simulink library "SUB_ECU_L4_MABX_HW_Interface"  (R2018a)
settings: Solver=VariableStepAuto  StartTime=0.0  StopTime=10.0  RelTol=1e-3
PostLoadFcn:
  | , if any(exist('dsrtsu_mdlpostloadfcn', 'file') == [2, 3, 6]), try dsrtsu_mdlpostloadfcn('Execute', bdroot); catch fprintf('Error in PostLoadFcn (dsrtsu_mdlpostloadfcn) for model "%s":\n %s\n', bdroot, lasterr); end, end,
undefined symbols (not defined in the file or in its folder): CANR_PROPB_REAX_3_13_CHANNEL_APV, CANR_PROPB_REAX_4_13_CHANNEL_APV, CANR_PROPB_XPR_1_50_CHANNEL_APV, ENUM_CAN_RX_T, ENUM_CAN_TX_T, ENUM_REAX_OPERATION_MODE_T, ENUM_SIGNAL_HEALTH_T, ENUM_XBR_CONTROL_MODE_T, ENUM_XBR_EBI_MODE_T, ENUM_XBR_PASS_THROUGH_ACTIVE_T, ENUM_XBR_PRIORITY_T, ENUM_XPR_INHIBIT_PARK_MANUAL_T, ENUM_XPR_INHIBIT_UNPARK_MANUAL_T, ENUM_XPR_PARK_MANUAL_T, ENUM_XPR_UNPARK_MANUAL_T, PROPB_REAX_1_E4_DES_POS_SIG_SRC_APV, PROPB_REAX_1_E4_DESIRED_OPMODE_APV, PROPB_REAX_1_E4_DESIRED_POSITION_APV, ptc_matlab_lib
libraries: PTC_MBDS_LIB x264, rtican x172, EmE_MBD_Blockset x39, simulink x34, $bdroot x16, rti1401lib_dio_type4 x8, simulink_need_slupdate x7, dsa_tcpip_lib x4, rti1401lib_adc_type4 x3, rtmapslib x3, rtitasklib x3
(part 17 of 51)

== system SUB_ECU_L4_MABX_HW_Interface/CAN_PIC_KW/CAN_RX_GNSSDOPs_00/RX_CAN_4 ==
  Enable : Inport
  Bus Creator1 : BusCreator  Inputs=9
  Bus Creator3 : BusCreator  Inputs=9
  Data Type Conversion{1..2,9..10} (4 alike) : DataTypeConversion  OutDataTypeStr=double  SaturateOnIntegerOverflow=on
  Data Type Conversion3 : DataTypeConversion  OutDataTypeStr=boolean  SaturateOnIntegerOverflow=on
  Data Type Conversion8 : DataTypeConversion  OutDataTypeStr=boolean  SaturateOnIntegerOverflow=on
  GNSSDOPs_011 : rtican/RTICAN Receive (RX)   Reserved1=[]  Reserved2=[]  Reserved3=[]  Reserved4=[]  SfcnMessage=[]  Msg_Struct=[]  BoardTypeNo=[]  BoardNo=[]  ChannelNo=[]  Parameters=[]  DialogFcn=[]  UnitName=[]  Revision=[]  UnitValues=[]  DSProperties=struct('RTI',struct('Version',uint32(5),'BlockType',struct('isSLSource',uint8(1),'isSLSink',uint8(1),'isHWSource',uint8(0),'isHWSink',uint8(0),'isSetup',uint8(0),'isInline',uint8(1),'isNonInline',uint8(0),'isInterrupt',uint8(0),'isChannelwise',uint8(0)),'IOBoardType','RTICAN','UnitType','MESSAGE','Identifier','RX','DialogType','MSVC','BlockSet','RTICAN','SlaveProcessor','CAN'))  RTIBlockInterface=struct('OutputPortsWidth',int32([1 1 1 1 1 1 1 1 1]),'OutputPortsActive',[1 1 1 1 1 1 1 1 1],'OutputPortsName',{{'SID','SetMode','OpMode','HDOP_','VDOP','TDOP',['RX status'],['RX time'],['RX delta time']}},'OutputPortsDataType',{{'SS_DOUBLE','SS_DOUBLE','SS_DOUBLE','SS_DOUBLE','SS_DOUBLE','SS_DOUBLE','SS_DOUBLE','SS_DOUBLE','SS_DOUBLE'}},'OutputPortsLabel',{{'SID','SetMode','OpMode','HDOP_','VDOP','TDOP','','',''}},'OutputPortsLabelMode','ON','InputPortsWidth',int32(0),'InputPortsActive',0,'DialogFcn','rtican_message_interface_gui','BlockDisplay',{{'','center'}},'IconTransparency','on','ParameterTunableNames',{{}},'InitLevel',3,'BlockName',struct('Token',{{'GNSSDOPs_01'}}),'SampleTime',{{-1}},'TriggerPort',{{'none'}},'EnablePort',{{'yes'}})  RTIBlockParameters=struct('BoardTypeNo',{{1,'OFF',[]}},'BoardNo',{{2,'ON',[1 16]}},'ChannelNo',{{2,'ON',[1 2]}},'Parameters',{{struct('DataFileSupport',struct('DataFileSelectedMaster',1,'DataFileSelectedLocal',0,'DataFileName','c:\localdata\chris\advanced_r&d\adas\level4_rcp\truck1571\dbc\mabx_can4.dbc|','DataFileDate',{{{['10-Feb-2017 15:17:28']}}},'SelectedFile','dbc\mabx_can4.dbc'),'Options',struct('StatusSelected',1,'TimeSelected',1,'DeltaTimeSelected',1,'BytePortSelected',0,'MessageLengthSelected',0,'TriggerPort',struct('Selected',0,'TriggerType',0),'UserCoding',struct('Selected',0,'InterfaceFile','UserDecodingFile','FcnName','UserDecodeFcn','InportSelected',0,'InportWidth',1,'OutportSelected',0,'OutportWidth',1),'EnablePortSelected',1,'SignalOnPortnameSelected',1,'UseRXService',1),'Message',struct('MsgOnBlocknameSelected',1,'MsgName','GNSSDOPs_01','MsgIdFormat',1,'MsgId',435815168,'MsgLength',8,'NumSignals',6,'SampleTime',-1,'Signal',struct('SgnName',{'SID','SetMode','OpMode','HDOP_','VDOP','TDOP'},'SgnStartBit',{0,8,11,16,32,48},'SgnLength',{8,3,3,16,16,16},'SgnType',{0,0,0,0,0,0},'ModeValue',{-1,-1,-1,-1,-1,-1},'DataType',{0,0,0,1,1,1},'ByteLayout',{0,0,0,0,0,0},'Factor',{1,1,1,0.01,0.01,0.01},'Offset',{0,0,0,0,0,0},'SgnComment',{{['An upward counting number used to tie related information together between different PGNs.For example,SID would be used to tie together COG,SOG and RAIM values to a given Pos.255=no valid Pos fix to tie it to.Range 0 to 250 for valid Pos fixes.']},{['0 = 1D, ' char(10) ' 1 = 2D, ' char(10) ' 2 = 3D, ' char(10) ' 3 = Auto, ' char(10) '4-5 = Reserved, ' char(10) ' 6 = Error, ' char(10) ' 7 = Null']},{['0 = 1D, ' char(10) ' 1 = 2D, ' char(10) ' 2 = 3D, ' char(10) ' 3 = Auto, ' char(10) '4-5 = Reserved, ' char(10) ' 6 = Error, ' char(10) ' 7 = Null']},{['Dilution of Precision(DOP)indicates contribution of satellite Config geometry to Posing error.A lower DOP value is preferred because less error is being introduced.Reported as components:HDOP(Horizontal),VDOP(Vertical),TDOP(Time).Min DOP value is 1.0(no e']},{['Dilution of Precision(DOP)indicates contribution of satellite Config geometry to Posing error.A lower DOP value is preferred because less error is being introduced.Reported as components:HDOP(Horizontal),VDOP(Vertical),TDOP(Time).Min DOP value is 1.0(no e']},{['Dilution of Precision(DOP)indicates contribution of satellite Config geometry to Posing error.A lower DOP value is preferred because less error is being introduced.Reported as components:HDOP(Horizontal),VDOP(Vertical),TDOP(Time).Min DOP value is 1.0(no e']}},'SgnUnit',{'','','','','',''},'Min',{0,0,0,-327.64,-327.64,-327.64},'Max',{252,7,7,327.64,327.64,327.64},'SLDataType',{'SS_DOUBLE','SS_DOUBLE','SS_DOUBLE','SS_DOUBLE','SS_DOUBLE','SS_DOUBLE'}),'MsgIdNumFormat',1,'MsgComment',{{['This PGN provides a single Trans containing GNSS status and dilution of precision components(DOP)that ']}}),'Version',1.2,'general',struct('isFromLib',0)),'OFF',[]}},'GroupId',{{struct('Group',{{'RTICAN'}},'No',28,'Behavior',{{'NAMECHANGE'}},'BlockType',{{'SINK'}},'NameChangeFlag',0),'OFF',[]}},'SFcnRTICANMessage',{{struct('MsgType','RX','SFcnPortType','Scalar','MsgName','GNSSDOPs_01','MsgIdFormat','XTD','MsgId',435815168,'MsgLength',8,'NumSignals',6,'SampleTime',-1,'Signal',struct('SgnName',{'SID','SetMode','OpMode','HDOP_','VDOP','TDOP'},'SgnStartBit',{0,8,11,16,32,48},'SgnLength',{8,3,3,16,16,16},'SgnType',{'standard','standard','standard','standard','standard','standard'},'ModeValue',{-1,-1,-1,-1,-1,-1},'DataType',{['unsigned int'],['unsigned int'],['unsigned int'],['signed int'],['signed int'],['signed int']},'ByteLayout',{['little endian'],['little endian'],['little endian'],['little endian'],['little endian'],['little endian']},'Factor',{1,1,1,0.01,0.01,0.01},'Offset',{0,0,0,0,0,0},'SLDataType',{'SS_DOUBLE','SS_DOUBLE','SS_DOUBLE','SS_DOUBLE','SS_DOUBLE','SS_DOUBLE'}),'StatusSelected','yes','TimeSelected','yes','DeltaTimeSelected','yes','BytePortSelected','no','MessageLengthSelected','no','TriggerPort',struct('Selected','no','TriggerType',0),'UserCoding',struct('Selected','no','InterfaceFile','UserDecodingFile','FcnName','UserDecodeFcn','InportSelected','no','InportWidth',1,'OutportSelected','no','OutportWidth',1),'EnablePortSelected','yes','UseRXService','yes','BoardType','DS1','BoardNo',2,'ControllerNo',2),'OFF',[]}},'TLCFileName',{{'rtican_rx_message','OFF',[]}})  RTISFcnParameters=struct('SFcnRTICANMessage','struct','TLCFileName','char')  RTIBlockParaDefault=struct('BoardTypeNo',4302,'BoardNo',1,'ChannelNo',1,'Parameters',struct('DataFileSupport',struct('DataFileSelectedMaster',0,'DataFileSelectedLocal',0,'DataFileName','','DataFileDate','','SelectedFile',['<no file selected>']),'Options',struct('StatusSelected',1,'TimeSelected',1,'DeltaTimeSelected',1,'BytePortSelected',0,'MessageLengthSelected',0,'TriggerPort',struct('Selected',0,'TriggerType','rising'),'UserCoding',struct('Selected',0,'InterfaceFile','UserDecodingFile','FcnName','UserDecodeFcn','InportSelected',0,'InportWidth',1,'OutportSelected',0,'OutportWidth',1),'EnablePortSelected',0,'SignalOnPortnameSelected',1,'UseRXService',0),'Message',struct('MsgOnBlocknameSelected',0,'MsgName',['RX Message'],'MsgIdFormat',0,'MsgId',100,'MsgLength',8,'NumSignals',1,'SampleTime',-1,'Signal',struct('SgnName',['RX signal'],'SgnStartBit',0,'SgnLength',8,'SgnType',0,'ModeValue',-1,'DataType',0,'SLDataType','SS_DOUBLE','ByteLayout',0,'Factor',1,'Offset',0,'Min',0,'Max',255,'SgnComment',{{}},'SgnUnit',''),'MsgIdNumFormat',0,'MsgComment',{{''}}),'Version',1.2,'general',struct('isFromLib',1)),'GroupId',struct('Group',{{'RTICAN'}},'No',1,'Behavior',{{'NAMECHANGE'}},'BlockType',{{'SINK'}},'NameChangeFlag',0),'SFcnRTICANMessage',struct('MsgType','RX','MsgName',['RX Message'],'MsgIdFormat','STD','MsgId',100,'MsgLength',8,'NumSignals',1,'SampleTime',-1,'Signal',struct('SgnName',['RX signal'],'SgnStartBit',0,'SgnLength',8,'SgnType','standard','ModeValue',-1,'DataType',['unsigned int'],'ByteLayout',['little endian'],'SLDataType','SS_DOUBLE','Factor',1,'Offset',0),'StatusSelected','yes','TimeSelected','yes','DeltaTimeSelected','yes','BytePortSelected','no','MessageLengthSelected','no','EnablePortSelected','no','UserCoding',struct('Selected','no','InterfaceFile','UserDecodingFile','FcnName','UserDecodeFcn','InportSelected','no','InportWidth',1,'OutportSelected','no','OutportWidth',1),'TriggerPort',struct('Selected','no','TriggerType','rising'),'UseRXService','no','BoardType','DS4302','BoardNo',1,'ControllerNo',1,'SFcnPortType','Scalar'),'TLCFileName','rtican_rx_message')
      settings: AttributesFormatString=Group Id: RTICAN28\n  SourceProductName=dSPACE RTI CAN Blockset
  GNSSDOPs_1 : rtican/RTICAN Receive (RX)   Reserved1=[]  Reserved2=[]  Reserved3=[]  Reserved4=[]  SfcnMessage=[]  Msg_Struct=[]  BoardTypeNo=[]  BoardNo=[]  ChannelNo=[]  Parameters=[]  DialogFcn=[]  UnitName=[]  Revision=[]  UnitValues=[]  DSProperties=struct('RTI',struct('Version',uint32(5),'BlockType',struct('isSLSource',uint8(1),'isSLSink',uint8(1),'isHWSource',uint8(0),'isHWSink',uint8(0),'isSetup',uint8(0),'isInline',uint8(1),'isNonInline',uint8(0),'isInterrupt',uint8(0),'isChannelwise',uint8(0)),'IOBoardType','RTICAN','UnitType','MESSAGE','Identifier','RX','DialogType','MSVC','BlockSet','RTICAN','SlaveProcessor','CAN'))  RTIBlockInterface=struct('OutputPortsWidth',int32([1 1 1 1 1 1 1 1 1]),'OutputPortsActive',[1 1 1 1 1 1 1 1 1],'OutputPortsName',{{'SID','SetMode','OpMode','HDOP_','VDOP','TDOP',['RX status'],['RX time'],['RX delta time']}},'OutputPortsDataType',{{'SS_DOUBLE','SS_DOUBLE','SS_DOUBLE','SS_DOUBLE','SS_DOUBLE','SS_DOUBLE','SS_DOUBLE','SS_DOUBLE','SS_DOUBLE'}},'OutputPortsLabel',{{'SID','SetMode','OpMode','HDOP_','VDOP','TDOP','','',''}},'OutputPortsLabelMode','ON','InputPortsWidth',int32(0),'InputPortsActive',0,'DialogFcn','rtican_message_interface_gui','BlockDisplay',{{'','center'}},'IconTransparency','on','ParameterTunableNames',{{}},'InitLevel',3,'BlockName',struct('Token',{{'GNSSDOPs_01'}}),'SampleTime',{{-1}},'TriggerPort',{{'none'}},'EnablePort',{{'yes'}})  RTIBlockParameters=struct('BoardTypeNo',{{1,'OFF',[]}},'BoardNo',{{2,'ON',[1 16]}},'ChannelNo',{{2,'ON',[1 2]}},'Parameters',{{struct('DataFileSupport',struct('DataFileSelectedMaster',1,'DataFileSelectedLocal',0,'DataFileName',['c:\localdata\chris\advanced_tech\adas\ptc_autonomous_truck_secure\branches\truck1571\dbc\mabx_can4.dbc|c:\localdata\chris\advanced_tech\adas\ptc_autonomous_truck_secure\branches\svn\powertrainsys\trunk\src\projects_rcp\my2017_rcp\dbc files\j1939.dbc|'],'DataFileDate',{{{['10-Feb-2017 15:17:28']}}},'SelectedFile',['<no file selected>']),'Options',struct('StatusSelected',1,'TimeSelected',1,'DeltaTimeSelected',1,'BytePortSelected',0,'MessageLengthSelected',0,'TriggerPort',struct('Selected',0,'TriggerType',0),'UserCoding',struct('Selected',0,'InterfaceFile','UserDecodingFile','FcnName','UserDecodeFcn','InportSelected',0,'InportWidth',1,'OutportSelected',0,'OutportWidth',1),'EnablePortSelected',1,'SignalOnPortnameSelected',1,'UseRXService',1),'Message',struct('MsgOnBlocknameSelected',1,'MsgName','GNSSDOPs_01','MsgIdFormat',1,'MsgId',435815169,'MsgLength',8,'NumSignals',6,'SampleTime',-1,'Signal',struct('SgnName',{'SID','SetMode','OpMode','HDOP_','VDOP','TDOP'},'SgnStartBit',{0,8,11,16,32,48},'SgnLength',{8,3,3,16,16,16},'SgnType',{0,0,0,0,0,0},'ModeValue',{-1,-1,-1,-1,-1,-1},'DataType',{0,0,0,1,1,1},'ByteLayout',{0,0,0,0,0,0},'Factor',{1,1,1,0.01,0.01,0.01},'Offset',{0,0,0,0,0,0},'SgnComment',{{['An upward counting number used to tie related information together between different PGNs.For example,SID would be used to tie together COG,SOG and RAIM values to a given Pos.255=no valid Pos fix to tie it to.Range 0 to 250 for valid Pos fixes.']},{['0 = 1D, ' char(10) ' 1 = 2D, ' char(10) ' 2 = 3D, ' char(10) ' 3 = Auto, ' char(10) '4-5 = Reserved, ' char(10) ' 6 = Error, ' char(10) ' 7 = Null']},{['0 = 1D, ' char(10) ' 1 = 2D, ' char(10) ' 2 = 3D, ' char(10) ' 3 = Auto, ' char(10) '4-5 = Reserved, ' char(10) ' 6 = Error, ' char(10) ' 7 = Null']},{['Dilution of Precision(DOP)indicates contribution of satellite Config geometry to Posing error.A lower DOP value is preferred because less error is being introduced.Reported as components:HDOP(Horizontal),VDOP(Vertical),TDOP(Time).Min DOP value is 1.0(no e']},{['Dilution of Precision(DOP)indicates contribution of satellite Config geometry to Posing error.A lower DOP value is preferred because less error is being introduced.Reported as components:HDOP(Horizontal),VDOP(Vertical),TDOP(Time).Min DOP value is 1.0(no e']},{['Dilution of Precision(DOP)indicates contribution of satellite Config geometry to Posing error.A lower DOP value is preferred because less error is being introduced.Reported as components:HDOP(Horizontal),VDOP(Vertical),TDOP(Time).Min DOP value is 1.0(no e']}},'SgnUnit',{'','','','','',''},'Min',{0,0,0,-327.64,-327.64,-327.64},'Max',{252,7,7,327.64,327.64,327.64},'SLDataType',{'SS_DOUBLE','SS_DOUBLE','SS_DOUBLE','SS_DOUBLE','SS_DOUBLE','SS_DOUBLE'}),'MsgIdNumFormat',1,'MsgComment',{{['This PGN provides a single Trans containing GNSS status and dilution of precision components(DOP)that ']}}),'Version',1.2,'general',struct('isFromLib',0)),'OFF',[]}},'GroupId',{{struct('Group',{{'RTICAN'}},'No',28,'Behavior',{{'NAMECHANGE'}},'BlockType',{{'SINK'}},'NameChangeFlag',0),'OFF',[]}},'SFcnRTICANMessage',{{struct('MsgType','RX','SFcnPortType','Scalar','MsgName','GNSSDOPs_01','MsgIdFormat','XTD','MsgId',435815169,'MsgLength',8,'NumSignals',6,'SampleTime',-1,'Signal',struct('SgnName',{'SID','SetMode','OpMode','HDOP_','VDOP','TDOP'},'SgnStartBit',{0,8,11,16,32,48},'SgnLength',{8,3,3,16,16,16},'SgnType',{'standard','standard','standard','standard','standard','standard'},'ModeValue',{-1,-1,-1,-1,-1,-1},'DataType',{['unsigned int'],['unsigned int'],['unsigned int'],['signed int'],['signed int'],['signed int']},'ByteLayout',{['little endian'],['little endian'],['little endian'],['little endian'],['little endian'],['little endian']},'Factor',{1,1,1,0.01,0.01,0.01},'Offset',{0,0,0,0,0,0},'SLDataType',{'SS_DOUBLE','SS_DOUBLE','SS_DOUBLE','SS_DOUBLE','SS_DOUBLE','SS_DOUBLE'}),'StatusSelected','yes','TimeSelected','yes','DeltaTimeSelected','yes','BytePortSelected','no','MessageLengthSelected','no','TriggerPort',struct('Selected','no','TriggerType',0),'UserCoding',struct('Selected','no','InterfaceFile','UserDecodingFile','FcnName','UserDecodeFcn','InportSelected','no','InportWidth',1,'OutportSelected','no','OutportWidth',1),'EnablePortSelected','yes','UseRXService','yes','BoardType','DS1','BoardNo',2,'ControllerNo',2),'OFF',[]}},'TLCFileName',{{'rtican_rx_message','OFF',[]}})  RTISFcnParameters=struct('SFcnRTICANMessage','struct','TLCFileName','char')  RTIBlockParaDefault=struct('BoardTypeNo',4302,'BoardNo',1,'ChannelNo',1,'Parameters',struct('DataFileSupport',struct('DataFileSelectedMaster',0,'DataFileSelectedLocal',0,'DataFileName','','DataFileDate','','SelectedFile',['<no file selected>']),'Options',struct('StatusSelected',1,'TimeSelected',1,'DeltaTimeSelected',1,'BytePortSelected',0,'MessageLengthSelected',0,'TriggerPort',struct('Selected',0,'TriggerType','rising'),'UserCoding',struct('Selected',0,'InterfaceFile','UserDecodingFile','FcnName','UserDecodeFcn','InportSelected',0,'InportWidth',1,'OutportSelected',0,'OutportWidth',1),'EnablePortSelected',0,'SignalOnPortnameSelected',1,'UseRXService',0),'Message',struct('MsgOnBlocknameSelected',0,'MsgName',['RX Message'],'MsgIdFormat',0,'MsgId',100,'MsgLength',8,'NumSignals',1,'SampleTime',-1,'Signal',struct('SgnName',['RX signal'],'SgnStartBit',0,'SgnLength',8,'SgnType',0,'ModeValue',-1,'DataType',0,'SLDataType','SS_DOUBLE','ByteLayout',0,'Factor',1,'Offset',0,'Min',0,'Max',255,'SgnComment',{{}},'SgnUnit',''),'MsgIdNumFormat',0,'MsgComment',{{''}}),'Version',1.2,'general',struct('isFromLib',1)),'GroupId',struct('Group',{{'RTICAN'}},'No',1,'Behavior',{{'NAMECHANGE'}},'BlockType',{{'SINK'}},'NameChangeFlag',0),'SFcnRTICANMessage',struct('MsgType','RX','MsgName',['RX Message'],'MsgIdFormat','STD','MsgId',100,'MsgLength',8,'NumSignals',1,'SampleTime',-1,'Signal',struct('SgnName',['RX signal'],'SgnStartBit',0,'SgnLength',8,'SgnType','standard','ModeValue',-1,'DataType',['unsigned int'],'ByteLayout',['little endian'],'SLDataType','SS_DOUBLE','Factor',1,'Offset',0),'StatusSelected','yes','TimeSelected','yes','DeltaTimeSelected','yes','BytePortSelected','no','MessageLengthSelected','no','EnablePortSelected','no','UserCoding',struct('Selected','no','InterfaceFile','UserDecodingFile','FcnName','UserDecodeFcn','InportSelected','no','InportWidth',1,'OutportSelected','no','OutportWidth',1),'TriggerPort',struct('Selected','no','TriggerType','rising'),'UseRXService','no','BoardType','DS4302','BoardNo',1,'ControllerNo',1,'SFcnPortType','Scalar'),'TLCFileName','rtican_rx_message')
      settings: AttributesFormatString=Group Id: RTICAN28\n  SourceProductName=dSPACE RTI CAN Blockset
  Switch : Switch  Criteria=u2 ~= 0
  GNSSDOPs_00 : Outport
  wires:
  GNSSDOPs_011/6 -> Bus Creator3/6  "TDOP"
  GNSSDOPs_011/5 -> Bus Creator3/5  "VDOP"
  GNSSDOPs_011/4 -> Bus Creator3/4  "HDOP_"
  GNSSDOPs_011/3 -> Bus Creator3/3  "OpMode"
  GNSSDOPs_011/2 -> Bus Creator3/2  "SetMode"
  GNSSDOPs_011/1 -> Bus Creator3/1  "SID"
  Bus Creator3/1 -> Switch/1  "GNSSDOPs_01"
  Enable/1 -> GNSSDOPs_1/Enable, GNSSDOPs_011/Enable
  GNSSDOPs_011/9 -> Data Type Conversion10/1
  GNSSDOPs_011/8 -> Data Type Conversion9/1
  GNSSDOPs_011/7 -> Data Type Conversion8/1
  Data Type Conversion8/1 -> Switch/2, Bus Creator3/7  "RX_status"
  Data Type Conversion10/1 -> Bus Creator3/9  "RX_delta_time"
  Data Type Conversion9/1 -> Bus Creator3/8  "RX_time"
  GNSSDOPs_1/6 -> Bus Creator1/6  "TDOP"
  Data Type Conversion3/1 -> Bus Creator1/7  "RX_status"
  Data Type Conversion1/1 -> Bus Creator1/9  "RX_delta_time"
  Data Type Conversion2/1 -> Bus Creator1/8  "RX_time"
  GNSSDOPs_1/4 -> Bus Creator1/4  "HDOP_"
  GNSSDOPs_1/5 -> Bus Creator1/5  "VDOP"
  GNSSDOPs_1/3 -> Bus Creator1/3  "OpMode"
  GNSSDOPs_1/2 -> Bus Creator1/2  "SetMode"
  GNSSDOPs_1/1 -> Bus Creator1/1  "SID"
  GNSSDOPs_1/7 -> Data Type Conversion3/1
  GNSSDOPs_1/8 -> Data Type Conversion2/1
  GNSSDOPs_1/9 -> Data Type Conversion1/1
  Bus Creator1/1 -> Switch/3
  Switch/1 -> GNSSDOPs_00/1

== system SUB_ECU_L4_MABX_HW_Interface/CAN_PIC_KW/CAN_RX_HRW_0B/RX_CAN_1 ==
  Enable : Inport
  Bus Creator3 : BusCreator  Inputs=7
  Data Type Conversion10 : DataTypeConversion  OutDataTypeStr=double  SaturateOnIntegerOverflow=on
  Data Type Conversion8 : DataTypeConversion  OutDataTypeStr=boolean  SaturateOnIntegerOverflow=on
  Data Type Conversion9 : DataTypeConversion  OutDataTypeStr=double  SaturateOnIntegerOverflow=on
  HRW_0B : rtican/RTICAN Receive (RX)   Reserved1=[]  Reserved2=[]  Reserved3=[]  Reserved4=[]  SfcnMessage=[]  Msg_Struct=[]  BoardTypeNo=[]  BoardNo=[]  ChannelNo=[]  Parameters=[]  DialogFcn=[]  UnitName=[]  Revision=[]  UnitValues=[]  DSProperties=struct('RTI',struct('Version',uint32(5),'BlockType',struct('isSLSource',uint8(1),'isSLSink',uint8(1),'isHWSource',uint8(0),'isHWSink',uint8(0),'isSetup',uint8(0),'isInline',uint8(1),'isNonInline',uint8(0),'isInterrupt',uint8(0),'isChannelwise',uint8(0)),'IOBoardType','RTICAN','UnitType','MESSAGE','Identifier','RX','DialogType','MSVC','BlockSet','RTICAN','SlaveProcessor','CAN'))  RTIBlockInterface=struct('OutputPortsWidth',int32([1 1 1 1 1 1 1]),'OutputPortsActive',[1 1 1 1 1 1 1],'OutputPortsName',{{'FrontAxleLeftWheelSpeed','FrontAxleRightWheelSpeed','RearAxleLeftWheelSpeed','RearAxleRightWheelSpeed',['RX status'],['RX time'],['RX delta time']}},'OutputPortsDataType',{{'SS_DOUBLE','SS_DOUBLE','SS_DOUBLE','SS_DOUBLE','SS_DOUBLE','SS_DOUBLE','SS_DOUBLE'}},'OutputPortsLabel',{{'FrontAxleLeftWheelSpeed','FrontAxleRightWheelSpeed','RearAxleLeftWheelSpeed','RearAxleRightWheelSpeed','','',''}},'OutputPortsLabelMode','ON','InputPortsWidth',int32(0),'InputPortsActive',0,'DialogFcn','rtican_message_interface_gui','BlockDisplay',{{'','center'}},'IconTransparency','on','ParameterTunableNames',{{}},'InitLevel',3,'BlockName',struct('Token',{{'HRW_0B'}}),'SampleTime',{{-1}},'TriggerPort',{{'none'}},'EnablePort',{{'yes'}})  RTIBlockParameters=struct('BoardTypeNo',{{1,'OFF',[]}},'BoardNo',{{1,'ON',[1 16]}},'ChannelNo',{{1,'ON',[1 2]}},'Parameters',{{struct('DataFileSupport',struct('DataFileSelectedMaster',1,'DataFileSelectedLocal',1,'DataFileName','c:\localdata\chris\advanced_tech\adas\level4_rcp\truck1571\dbc\j1939_famosdbcwithfusion.dbc|','DataFileDate',{{{['03-Apr-2017 12:55:40']}}},'SelectedFile','dbc\j1939_famosdbcwithfusion.dbc','InterfaceFcn','rtican_dbc_file_parser'),'Options',struct('StatusSelected',1,'TimeSelected',1,'DeltaTimeSelected',1,'BytePortSelected',0,'MessageLengthSelected',0,'TriggerPort',struct('Selected',0,'TriggerType',0),'UserCoding',struct('Selected',0,'InterfaceFile','UserDecodingFile','FcnName','UserDecodeFcn','InportSelected',0,'InportWidth',1,'OutportSelected',0,'OutportWidth',1),'EnablePortSelected',1,'SignalOnPortnameSelected',1,'UseRXService',1),'Message',struct('MsgOnBlocknameSelected',1,'MsgName','HRW_0B','MsgIdFormat',1,'MsgId',150892043,'MsgLength',8,'NumSignals',4,'SampleTime',-1,'Signal',struct('SgnName',{'FrontAxleLeftWheelSpeed','FrontAxleRightWheelSpeed','RearAxleLeftWheelSpeed','RearAxleRightWheelSpeed'},'SgnStartBit',{0,16,32,48},'SgnLength',{16,16,16,16},'SgnType',{0,0,0,0},'ModeValue',{-1,-1,-1,-1},'DataType',{0,0,0,0},'ByteLayout',{0,0,0,0},'Factor',{2^-8,2^-8,2^-8,2^-8},'Offset',{0,0,0,0},'SgnComment',{{['High resolution measurement of the speed of the left wheel on the front axle.']},{['High resolution measurement of the speed of the right wheel on the front axle.']},{['High resolution measurement of the speed of the left wheel on the rear axle.']},{['High resolution measurement of the speed of the right wheel on the rear axle.']}},'SgnUnit',{'km/h','km/h','km/h','km/h'},'Min',{0,0,0,0},'Max',{250.996,250.996,250.996,250.996},'SLDataType',{'SS_DOUBLE','SS_DOUBLE','SS_DOUBLE','SS_DOUBLE'}),'MsgIdNumFormat',0,'MsgComment',{{['High Resolution Wheel Speed']}}),'Version',1.2,'general',struct('isFromLib',0)),'OFF',[]}},'GroupId',{{struct('Group',{{'RTICAN'}},'No',25,'Behavior',{{'NAMECHANGE'}},'BlockType',{{'SINK'}},'NameChangeFlag',0),'OFF',[]}},'SFcnRTICANMessage',{{struct('MsgType','RX','SFcnPortType','Scalar','MsgName','HRW_0B','MsgIdFormat','XTD','MsgId',150892043,'MsgLength',8,'NumSignals',4,'SampleTime',-1,'Signal',struct('SgnName',{'FrontAxleLeftWheelSpeed','FrontAxleRightWheelSpeed','RearAxleLeftWheelSpeed','RearAxleRightWheelSpeed'},'SgnStartBit',{0,16,32,48},'SgnLength',{16,16,16,16},'SgnType',{'standard','standard','standard','standard'},'ModeValue',{-1,-1,-1,-1},'DataType',{['unsigned int'],['unsigned int'],['unsigned int'],['unsigned int']},'ByteLayout',{['little endian'],['little endian'],['little endian'],['little endian']},'Factor',{2^-8,2^-8,2^-8,2^-8},'Offset',{0,0,0,0},'SLDataType',{'SS_DOUBLE','SS_DOUBLE','SS_DOUBLE','SS_DOUBLE'}),'StatusSelected','yes','TimeSelected','yes','DeltaTimeSelected','yes','BytePortSelected','no','MessageLengthSelected','no','TriggerPort',struct('Selected','no','TriggerType',0),'UserCoding',struct('Selected','no','InterfaceFile','UserDecodingFile','FcnName','UserDecodeFcn','InportSelected','no','InportWidth',1,'OutportSelected','no','OutportWidth',1),'EnablePortSelected','yes','UseRXService','yes','BoardType','DS1','BoardNo',1,'ControllerNo',1),'OFF',[]}},'TLCFileName',{{'rtican_rx_message','OFF',[]}})  RTISFcnParameters=struct('SFcnRTICANMessage','struct','TLCFileName','char')  RTIBlockParaDefault=struct('BoardTypeNo',4302,'BoardNo',1,'ChannelNo',1,'Parameters',struct('DataFileSupport',struct('DataFileSelectedMaster',0,'DataFileSelectedLocal',0,'DataFileName','','DataFileDate','','SelectedFile',['<no file selected>']),'Options',struct('StatusSelected',1,'TimeSelected',1,'DeltaTimeSelected',1,'BytePortSelected',0,'MessageLengthSelected',0,'TriggerPort',struct('Selected',0,'TriggerType','rising'),'UserCoding',struct('Selected',0,'InterfaceFile','UserDecodingFile','FcnName','UserDecodeFcn','InportSelected',0,'InportWidth',1,'OutportSelected',0,'OutportWidth',1),'EnablePortSelected',0,'SignalOnPortnameSelected',1,'UseRXService',0),'Message',struct('MsgOnBlocknameSelected',0,'MsgName',['RX Message'],'MsgIdFormat',0,'MsgId',100,'MsgLength',8,'NumSignals',1,'SampleTime',-1,'Signal',struct('SgnName',['RX signal'],'SgnStartBit',0,'SgnLength',8,'SgnType',0,'ModeValue',-1,'DataType',0,'SLDataType','SS_DOUBLE','ByteLayout',0,'Factor',1,'Offset',0,'Min',0,'Max',255,'SgnComment',{{}},'SgnUnit',''),'MsgIdNumFormat',0,'MsgComment',{{''}}),'Version',1.2,'general',struct('isFromLib',1)),'GroupId',struct('Group',{{'RTICAN'}},'No',1,'Behavior',{{'NAMECHANGE'}},'BlockType',{{'SINK'}},'NameChangeFlag',0),'SFcnRTICANMessage',struct('MsgType','RX','MsgName',['RX Message'],'MsgIdFormat','STD','MsgId',100,'MsgLength',8,'NumSignals',1,'SampleTime',-1,'Signal',struct('SgnName',['RX signal'],'SgnStartBit',0,'SgnLength',8,'SgnType','standard','ModeValue',-1,'DataType',['unsigned int'],'ByteLayout',['little endian'],'SLDataType','SS_DOUBLE','Factor',1,'Offset',0),'StatusSelected','yes','TimeSelected','yes','DeltaTimeSelected','yes','BytePortSelected','no','MessageLengthSelected','no','EnablePortSelected','no','UserCoding',struct('Selected','no','InterfaceFile','UserDecodingFile','FcnName','UserDecodeFcn','InportSelected','no','InportWidth',1,'OutportSelected','no','OutportWidth',1),'TriggerPort',struct('Selected','no','TriggerType','rising'),'UseRXService','no','BoardType','DS4302','BoardNo',1,'ControllerNo',1,'SFcnPortType','Scalar'),'TLCFileName','rtican_rx_message')
      settings: AttributesFormatString=Group Id: RTICAN25\n  SourceProductName=dSPACE RTI CAN Blockset
  HRW_0B_ : Outport
  wires:
  HRW_0B/4 -> Bus Creator3/4  "RearAxleRightWheelSpeed"
  HRW_0B/3 -> Bus Creator3/3  "RearAxleLeftWheelSpeed"
  HRW_0B/2 -> Bus Creator3/2  "FrontAxleRightWheelSpeed"
  HRW_0B/1 -> Bus Creator3/1  "FrontAxleLeftWheelSpeed"
  Bus Creator3/1 -> HRW_0B_/1  "HRW_0B"
  Enable/1 -> HRW_0B/Enable
  HRW_0B/7 -> Data Type Conversion10/1
  HRW_0B/6 -> Data Type Conversion9/1
  HRW_0B/5 -> Data Type Conversion8/1
  Data Type Conversion8/1 -> Bus Creator3/5  "RX_status"
  Data Type Conversion10/1 -> Bus Creator3/7  "RX_delta_time"
  Data Type Conversion9/1 -> Bus Creator3/6  "RX_time"

== system SUB_ECU_L4_MABX_HW_Interface/CAN_PIC_KW/CAN_RX_PROPB_REAX_2_13/RX_CAN_4 ==
  Enable : Inport
  Bus Creator3 : BusCreator  Inputs=5
  Data Type Conversion10 : DataTypeConversion  OutDataTypeStr=double  SaturateOnIntegerOverflow=on
  Data Type Conversion8 : DataTypeConversion  OutDataTypeStr=boolean  SaturateOnIntegerOverflow=on
  Data Type Conversion9 : DataTypeConversion  OutDataTypeStr=double  SaturateOnIntegerOverflow=on
  PropB_REAX_2_13 : rtican/RTICAN Receive (RX)   Reserved1=[]  Reserved2=[]  Reserved3=[]  Reserved4=[]  SfcnMessage=[]  Msg_Struct=[]  BoardTypeNo=[]  BoardNo=[]  ChannelNo=[]  Parameters=[]  DialogFcn=[]  UnitName=[]  Revision=[]  UnitValues=[]  DSProperties=struct('RTI',struct('Version',uint32(5),'BlockType',struct('isSLSource',uint8(1),'isSLSink',uint8(1),'isHWSource',uint8(0),'isHWSink',uint8(0),'isSetup',uint8(0),'isInline',uint8(1),'isNonInline',uint8(0),'isInterrupt',uint8(0),'isChannelwise',uint8(0)),'IOBoardType','RTICAN','UnitType','MESSAGE','Identifier','RX','DialogType','MSVC','BlockSet','RTICAN','SlaveProcessor','CAN'))  RTIBlockInterface=struct('OutputPortsWidth',int32([1 1 1 1 1]),'OutputPortsActive',[1 1 1 1 1],'OutputPortsName',{{'PropB_REAX_2_ActualHandwheelPos','PropB_REAX_2_EchoedStrWhlPos',['RX status'],['RX time'],['RX delta time']}},'OutputPortsDataType',{{'SS_DOUBLE','SS_DOUBLE','SS_DOUBLE','SS_DOUBLE','SS_DOUBLE'}},'OutputPortsLabel',{{'PropB_REAX_2_ActualHandwheelPos','PropB_REAX_2_EchoedStrWhlPos','','',''}},'OutputPortsLabelMode','ON','InputPortsWidth',int32(0),'InputPortsActive',0,'DialogFcn','rtican_message_interface_gui','BlockDisplay',{{'','center'}},'IconTransparency','on','ParameterTunableNames',{{}},'InitLevel',3,'BlockName',struct('Token',{{'PropB_REAX_2_13'}}),'SampleTime',{{-1}},'TriggerPort',{{'none'}},'EnablePort',{{'yes'}})  RTIBlockParameters=struct('BoardTypeNo',{{1,'OFF',[]}},'BoardNo',{{2,'ON',[1 16]}},'ChannelNo',{{2,'ON',[1 2]}},'Parameters',{{struct('DataFileSupport',struct('DataFileSelectedMaster',1,'DataFileSelectedLocal',1,'DataFileName',['c:\localdata\chris\advanced_tech\adas\ptc_autonomous_truck_secure\branches\truck1571\dbc\mabx_can4.dbc|c:\localdata\chris\advanced_tech\adas\ptc_autonomous_truck_secure\branches\svn\powertrainsys\trunk\src\projects_rcp\my2017_rcp\dbc files\j1939.dbc|'],'DataFileDate',{{{['02-May-2017 14:24:53']},{['10-Feb-2017 15:17:28']}}},'SelectedFile','dbc\mabx_can4.dbc'),'Options',struct('StatusSelected',1,'TimeSelected',1,'DeltaTimeSelected',1,'BytePortSelected',0,'MessageLengthSelected',0,'TriggerPort',struct('Selected',0,'TriggerType',0),'UserCoding',struct('Selected',0,'InterfaceFile','UserDecodingFile','FcnName','UserDecodeFcn','InportSelected',0,'InportWidth',1,'OutportSelected',0,'OutportWidth',1),'EnablePortSelected',1,'SignalOnPortnameSelected',1,'UseRXService',1),'Message',struct('MsgOnBlocknameSelected',1,'MsgName','PropB_REAX_2_13','MsgIdFormat',1,'MsgId',419426323,'MsgLength',8,'NumSignals',2,'SampleTime',-1,'Signal',struct('SgnName',{'PropB_REAX_2_ActualHandwheelPos','PropB_REAX_2_EchoedStrWhlPos'},'SgnStartBit',{0,32},'SgnLength',{32,32},'SgnType',{0,0},'ModeValue',{-1,-1},'DataType',{1,1},'ByteLayout',{0,0},'Factor',{0.0439453125,0.0439453125},'Offset',{0,0},'SgnComment',{{['Actual handwheel position']},{['Echoed steering wheel position']}},'SgnUnit',{'deg','deg'},'Min',{0,0},'Max',{0,0},'SLDataType',{'SS_DOUBLE','SS_DOUBLE'}),'MsgIdNumFormat',0,'MsgComment',{{['Response message A from TRW steering wheel']}}),'Version',1.2,'general',struct('isFromLib',0)),'OFF',[]}},'GroupId',{{struct('Group',{{'RTICAN'}},'No',28,'Behavior',{{'NAMECHANGE'}},'BlockType',{{'SINK'}},'NameChangeFlag',0),'OFF',[]}},'SFcnRTICANMessage',{{struct('MsgType','RX','SFcnPortType','Scalar','MsgName','PropB_REAX_2_13','MsgIdFormat','XTD','MsgId',419426323,'MsgLength',8,'NumSignals',2,'SampleTime',-1,'Signal',struct('SgnName',{'PropB_REAX_2_ActualHandwheelPos','PropB_REAX_2_EchoedStrWhlPos'},'SgnStartBit',{0,32},'SgnLength',{32,32},'SgnType',{'standard','standard'},'ModeValue',{-1,-1},'DataType',{['signed int'],['signed int']},'ByteLayout',{['little endian'],['little endian']},'Factor',{0.0439453125,0.0439453125},'Offset',{0,0},'SLDataType',{'SS_DOUBLE','SS_DOUBLE'}),'StatusSelected','yes','TimeSelected','yes','DeltaTimeSelected','yes','BytePortSelected','no','MessageLengthSelected','no','TriggerPort',struct('Selected','no','TriggerType',0),'UserCoding',struct('Selected','no','InterfaceFile','UserDecodingFile','FcnName','UserDecodeFcn','InportSelected','no','InportWidth',1,'OutportSelected','no','OutportWidth',1),'EnablePortSelected','yes','UseRXService','yes','BoardType','DS1','BoardNo',3,'ControllerNo',1),'OFF',[]}},'TLCFileName',{{'rtican_rx_message','OFF',[]}})  RTISFcnParameters=struct('SFcnRTICANMessage','struct','TLCFileName','char')  RTIBlockParaDefault=struct('BoardTypeNo',4302,'BoardNo',1,'ChannelNo',1,'Parameters',struct('DataFileSupport',struct('DataFileSelectedMaster',0,'DataFileSelectedLocal',0,'DataFileName','','DataFileDate','','SelectedFile',['<no file selected>']),'Options',struct('StatusSelected',1,'TimeSelected',1,'DeltaTimeSelected',1,'BytePortSelected',0,'MessageLengthSelected',0,'TriggerPort',struct('Selected',0,'TriggerType','rising'),'UserCoding',struct('Selected',0,'InterfaceFile','UserDecodingFile','FcnName','UserDecodeFcn','InportSelected',0,'InportWidth',1,'OutportSelected',0,'OutportWidth',1),'EnablePortSelected',0,'SignalOnPortnameSelected',1,'UseRXService',0),'Message',struct('MsgOnBlocknameSelected',0,'MsgName',['RX Message'],'MsgIdFormat',0,'MsgId',100,'MsgLength',8,'NumSignals',1,'SampleTime',-1,'Signal',struct('SgnName',['RX signal'],'SgnStartBit',0,'SgnLength',8,'SgnType',0,'ModeValue',-1,'DataType',0,'SLDataType','SS_DOUBLE','ByteLayout',0,'Factor',1,'Offset',0,'Min',0,'Max',255,'SgnComment',{{}},'SgnUnit',''),'MsgIdNumFormat',0,'MsgComment',{{''}}),'Version',1.2,'general',struct('isFromLib',1)),'GroupId',struct('Group',{{'RTICAN'}},'No',1,'Behavior',{{'NAMECHANGE'}},'BlockType',{{'SINK'}},'NameChangeFlag',0),'SFcnRTICANMessage',struct('MsgType','RX','MsgName',['RX Message'],'MsgIdFormat','STD','MsgId',100,'MsgLength',8,'NumSignals',1,'SampleTime',-1,'Signal',struct('SgnName',['RX signal'],'SgnStartBit',0,'SgnLength',8,'SgnType','standard','ModeValue',-1,'DataType',['unsigned int'],'ByteLayout',['little endian'],'SLDataType','SS_DOUBLE','Factor',1,'Offset',0),'StatusSelected','yes','TimeSelected','yes','DeltaTimeSelected','yes','BytePortSelected','no','MessageLengthSelected','no','EnablePortSelected','no','UserCoding',struct('Selected','no','InterfaceFile','UserDecodingFile','FcnName','UserDecodeFcn','InportSelected','no','InportWidth',1,'OutportSelected','no','OutportWidth',1),'TriggerPort',struct('Selected','no','TriggerType','rising'),'UseRXService','no','BoardType','DS4302','BoardNo',1,'ControllerNo',1,'SFcnPortType','Scalar'),'TLCFileName','rtican_rx_message')
      settings: AttributesFormatString=Group Id: RTICAN28\n  SourceProductName=dSPACE RTI CAN Blockset
  PROPB_REAX_2_13 : Outport
  wires:
  Bus Creator3/1 -> PROPB_REAX_2_13/1  "PROPB_REAX_2_13"
  Enable/1 -> PropB_REAX_2_13/Enable
  PropB_REAX_2_13/5 -> Data Type Conversion10/1
  PropB_REAX_2_13/4 -> Data Type Conversion9/1
  PropB_REAX_2_13/3 -> Data Type Conversion8/1
  Data Type Conversion8/1 -> Bus Creator3/3  "RX_status"
  Data Type Conversion10/1 -> Bus Creator3/5  "RX_delta_time"
  Data Type Conversion9/1 -> Bus Creator3/4  "RX_time"
  PropB_REAX_2_13/1 -> Bus Creator3/1  "PropB_REAX_2_ActualHandwheelPos"
  PropB_REAX_2_13/2 -> Bus Creator3/2  "PropB_REAX_2_EchoedStrWhlPos"

== system SUB_ECU_L4_MABX_HW_Interface/CAN_PIC_KW/CAN_RX_PROPB_REAX_2_13/RX_CAN_5 ==
  Enable : Inport
  Bus Creator3 : BusCreator  Inputs=5
  Data Type Conversion10 : DataTypeConversion  OutDataTypeStr=double  SaturateOnIntegerOverflow=on
  Data Type Conversion8 : DataTypeConversion  OutDataTypeStr=boolean  SaturateOnIntegerOverflow=on
  Data Type Conversion9 : DataTypeConversion  OutDataTypeStr=double  SaturateOnIntegerOverflow=on
  PropB_REAX_2_13 : rtican/RTICAN Receive (RX)   Reserved1=[]  Reserved2=[]  Reserved3=[]  Reserved4=[]  SfcnMessage=[]  Msg_Struct=[]  BoardTypeNo=[]  BoardNo=[]  ChannelNo=[]  Parameters=[]  DialogFcn=[]  UnitName=[]  Revision=[]  UnitValues=[]  DSProperties=struct('RTI',struct('Version',uint32(5),'BlockType',struct('isSLSource',uint8(1),'isSLSink',uint8(1),'isHWSource',uint8(0),'isHWSink',uint8(0),'isSetup',uint8(0),'isInline',uint8(1),'isNonInline',uint8(0),'isInterrupt',uint8(0),'isChannelwise',uint8(0)),'IOBoardType','RTICAN','UnitType','MESSAGE','Identifier','RX','DialogType','MSVC','BlockSet','RTICAN','SlaveProcessor','CAN'))  RTIBlockInterface=struct('OutputPortsWidth',int32([1 1 1 1 1]),'OutputPortsActive',[1 1 1 1 1],'OutputPortsName',{{'PropB_REAX_2_ActualHandwheelPos','PropB_REAX_2_EchoedStrWhlPos',['RX status'],['RX time'],['RX delta time']}},'OutputPortsDataType',{{'SS_DOUBLE','SS_DOUBLE','SS_DOUBLE','SS_DOUBLE','SS_DOUBLE'}},'OutputPortsLabel',{{'PropB_REAX_2_ActualHandwheelPos','PropB_REAX_2_EchoedStrWhlPos','','',''}},'OutputPortsLabelMode','ON','InputPortsWidth',int32(0),'InputPortsActive',0,'DialogFcn','rtican_message_interface_gui','BlockDisplay',{{'','center'}},'IconTransparency','on','ParameterTunableNames',{{}},'InitLevel',3,'BlockName',struct('Token',{{'PropB_REAX_2_13'}}),'SampleTime',{{-1}},'TriggerPort',{{'none'}},'EnablePort',{{'yes'}})  RTIBlockParameters=struct('BoardTypeNo',{{1,'OFF',[]}},'BoardNo',{{3,'ON',[1 16]}},'ChannelNo',{{1,'ON',[1 2]}},'Parameters',{{struct('DataFileSupport',struct('DataFileSelectedMaster',1,'DataFileSelectedLocal',1,'DataFileName','c:\dev\svn\adv_adas_shared\branches\sundeep.tuteja\project_l4\src\dbc\mabx_can4_chrisbaltonallstandard.dbc|c:\dev\svn\adv_adas_shared\branches\sundeep.tuteja\project_l4\src\dbc\mabx_can4.dbc|','DataFileDate',{{{['02-May-2017 14:24:53']},{['10-Feb-2017 15:17:28']}}},'SelectedFile','dbc\mabx_can4.dbc'),'Options',struct('StatusSelected',1,'TimeSelected',1,'DeltaTimeSelected',1,'BytePortSelected',0,'MessageLengthSelected',0,'TriggerPort',struct('Selected',0,'TriggerType',0),'UserCoding',struct('Selected',0,'InterfaceFile','UserDecodingFile','FcnName','UserDecodeFcn','InportSelected',0,'InportWidth',1,'OutportSelected',0,'OutportWidth',1),'EnablePortSelected',1,'SignalOnPortnameSelected',1,'UseRXService',1),'Message',struct('MsgOnBlocknameSelected',1,'MsgName','PropB_REAX_2_13','MsgIdFormat',1,'MsgId',419426323,'MsgLength',8,'NumSignals',2,'SampleTime',-1,'Signal',struct('SgnName',{'PropB_REAX_2_ActualHandwheelPos','PropB_REAX_2_EchoedStrWhlPos'},'SgnStartBit',{0,32},'SgnLength',{32,32},'SgnType',{0,0},'ModeValue',{-1,-1},'DataType',{1,1},'ByteLayout',{0,0},'Factor',{0.0439453125,0.0439453125},'Offset',{0,0},'SgnComment',{{['Actual handwheel position']},{['Echoed steering wheel position']}},'SgnUnit',{'deg','deg'},'Min',{0,0},'Max',{0,0},'SLDataType',{'SS_DOUBLE','SS_DOUBLE'}),'MsgIdNumFormat',1,'MsgComment',{{['Response message A from TRW steering wheel']}}),'Version',1.2,'general',struct('isFromLib',0)),'OFF',[]}},'GroupId',{{struct('Group',{{'RTICAN'}},'No',29,'Behavior',{{'NAMECHANGE'}},'BlockType',{{'SINK'}},'NameChangeFlag',0),'OFF',[]}},'SFcnRTICANMessage',{{struct('MsgType','RX','SFcnPortType','Scalar','MsgName','PropB_REAX_2_13','MsgIdFormat','XTD','MsgId',419426323,'MsgLength',8,'NumSignals',2,'SampleTime',-1,'Signal',struct('SgnName',{'PropB_REAX_2_ActualHandwheelPos','PropB_REAX_2_EchoedStrWhlPos'},'SgnStartBit',{0,32},'SgnLength',{32,32},'SgnType',{'standard','standard'},'ModeValue',{-1,-1},'DataType',{['signed int'],['signed int']},'ByteLayout',{['little endian'],['little endian']},'Factor',{0.0439453125,0.0439453125},'Offset',{0,0},'SLDataType',{'SS_DOUBLE','SS_DOUBLE'}),'StatusSelected','yes','TimeSelected','yes','DeltaTimeSelected','yes','BytePortSelected','no','MessageLengthSelected','no','TriggerPort',struct('Selected','no','TriggerType',0),'UserCoding',struct('Selected','no','InterfaceFile','UserDecodingFile','FcnName','UserDecodeFcn','InportSelected','no','InportWidth',1,'OutportSelected','no','OutportWidth',1),'EnablePortSelected','yes','UseRXService','yes','BoardType','DS1','BoardNo',3,'ControllerNo',1),'OFF',[]}},'TLCFileName',{{'rtican_rx_message','OFF',[]}})  RTISFcnParameters=struct('SFcnRTICANMessage','struct','TLCFileName','char')  RTIBlockParaDefault=struct('BoardTypeNo',4302,'BoardNo',1,'ChannelNo',1,'Parameters',struct('DataFileSupport',struct('DataFileSelectedMaster',0,'DataFileSelectedLocal',0,'DataFileName','','DataFileDate','','SelectedFile',['<no file selected>']),'Options',struct('StatusSelected',1,'TimeSelected',1,'DeltaTimeSelected',1,'BytePortSelected',0,'MessageLengthSelected',0,'TriggerPort',struct('Selected',0,'TriggerType','rising'),'UserCoding',struct('Selected',0,'InterfaceFile','UserDecodingFile','FcnName','UserDecodeFcn','InportSelected',0,'InportWidth',1,'OutportSelected',0,'OutportWidth',1),'EnablePortSelected',0,'SignalOnPortnameSelected',1,'UseRXService',0),'Message',struct('MsgOnBlocknameSelected',0,'MsgName',['RX Message'],'MsgIdFormat',0,'MsgId',100,'MsgLength',8,'NumSignals',1,'SampleTime',-1,'Signal',struct('SgnName',['RX signal'],'SgnStartBit',0,'SgnLength',8,'SgnType',0,'ModeValue',-1,'DataType',0,'SLDataType','SS_DOUBLE','ByteLayout',0,'Factor',1,'Offset',0,'Min',0,'Max',255,'SgnComment',{{}},'SgnUnit',''),'MsgIdNumFormat',0,'MsgComment',{{''}}),'Version',1.2,'general',struct('isFromLib',1)),'GroupId',struct('Group',{{'RTICAN'}},'No',1,'Behavior',{{'NAMECHANGE'}},'BlockType',{{'SINK'}},'NameChangeFlag',0),'SFcnRTICANMessage',struct('MsgType','RX','MsgName',['RX Message'],'MsgIdFormat','STD','MsgId',100,'MsgLength',8,'NumSignals',1,'SampleTime',-1,'Signal',struct('SgnName',['RX signal'],'SgnStartBit',0,'SgnLength',8,'SgnType','standard','ModeValue',-1,'DataType',['unsigned int'],'ByteLayout',['little endian'],'SLDataType','SS_DOUBLE','Factor',1,'Offset',0),'StatusSelected','yes','TimeSelected','yes','DeltaTimeSelected','yes','BytePortSelected','no','MessageLengthSelected','no','EnablePortSelected','no','UserCoding',struct('Selected','no','InterfaceFile','UserDecodingFile','FcnName','UserDecodeFcn','InportSelected','no','InportWidth',1,'OutportSelected','no','OutportWidth',1),'TriggerPort',struct('Selected','no','TriggerType','rising'),'UseRXService','no','BoardType','DS4302','BoardNo',1,'ControllerNo',1,'SFcnPortType','Scalar'),'TLCFileName','rtican_rx_message')
      settings: AttributesFormatString=Group Id: RTICAN29\n  SourceProductName=dSPACE RTI CAN Blockset
  PROPB_REAX_2_13 : Outport
  wires:
  PropB_REAX_2_13/2 -> Bus Creator3/2  "PropB_REAX_2_EchoedStrWhlPos"
  PropB_REAX_2_13/1 -> Bus Creator3/1  "PropB_REAX_2_ActualHandwheelPos"
  Data Type Conversion9/1 -> Bus Creator3/4  "RX_time"
  Data Type Conversion10/1 -> Bus Creator3/5  "RX_delta_time"
  Data Type Conversion8/1 -> Bus Creator3/3  "RX_status"
  PropB_REAX_2_13/3 -> Data Type Conversion8/1
  PropB_REAX_2_13/4 -> Data Type Conversion9/1
  PropB_REAX_2_13/5 -> Data Type Conversion10/1
  Enable/1 -> PropB_REAX_2_13/Enable
  Bus Creator3/1 -> PROPB_REAX_2_13/1  "PROPB_REAX_2_13"
